simulink model "PID_AW_d"  (R2015b)
settings: Solver=VariableStepAuto  StartTime=0.0  StopTime=10.0  RelTol=1e-3
undefined symbols (not defined in the file): D_d, I_d, P_d, sat_lim_max, sat_lim_min, timestep
settings Model: Creator=mgreiff  LastModifiedBy=mgreiff

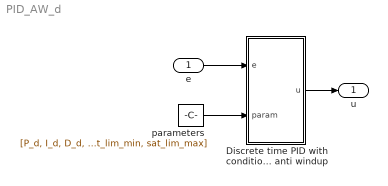
== system PID_AW_d ==
  e : Inport
  Discrete time PID with conditional anti windup : MATLAB Function  TreatAsAtomicUnit=on
  parameters : Constant  Value=[P_d, I_d, D_d, timestep, sat_lim_min, sat_lim_max]
  u : Outport
  wires:
  e/1 -> Discrete time PID with conditional anti windup/1(e)
  Discrete time PID with conditional anti windup/1(u) -> u/1
  parameters/1 -> Discrete time PID with conditional anti windup/2(param)

== matlab function PID_AW_d/Discrete time PID with conditional anti windup ==
  data: e input; u output; param input
function u = PID_AW_d(e, param)
%#codegen
Kp = param(1); Ki = param(2); Kd = param(3); h = param(4);
sat_lim_max = param(5); sat_lim_min = param(6); 
persistent I
persistent em1
persistent um1
if isempty(I) || isempty(em1)
    I = 0; em1 = 0; um1 = 0;
end
P = Kp * e;
if um1 <= sat_lim_max && um1 >= sat_lim_min
    I = I + Ki * h * e;
end
D = Kd * (e - em1)/h;
em1 = e;
u = P + I + D;
